simulink model "IndirectKalmanFilter"  (R2023b)
settings: Solver=ode4  StartTime=0.0  StopTime=2800  FixedStep=filter_Ts  RelTol=1e-3
InitFcn:
  | loadData;
values from neighbouring files (symbols this model uses):
  B_0 = Bk(x_0, imuSim.signals.values(1, 1:3)', imuSim.signals.values(1, 4:6)', filter_Ts)    [loadData.m]
  dx_0 = zeros(length(x_0), 1)    [loadData.m]
  F_0 = Fk(x_0, imuSim.signals.values(1, 1:3)', imuSim.signals.values(1, 4:6)', filter_Ts)    [loadData.m]
  filter_Ts = 0.01    [loadData.m]
  gps_sampling_time = 0.1    [loadData.m]
  imu_sampling_time = 0.01    [loadData.m]
  p_0 = 100 * eye(9)    [loadData.m]
  Qk = diag([1e-10, 1e-10, 1e-10, accel_var_continuous, gyro_var_continuous])    [computeImuProcessNoise.m]    (also in loadData.m = diag([1e-11, 1e-11, 1e-11, 4e-5,  4e-5,  4e-5, 1.2e-5, 1.2e-)
  Rk = diag([(7.84e-5)^2, (7.84e-5)^2, (2.0)^2, (0.1)^2, (0.1)^2, (0.1)^2])    [loadData.m]
  u_0 = imuSim.signals.values(1, :)    [loadData.m]
  x_0 = [lon_0;lat_0;h_0;vn_0;ve_0;vd_0;phi_0;theta_0;si_0]    [loadData.m]
libraries: simulink_extras x6, matrix_library x1
settings Model: Creator=amir  LastModifiedBy=amir

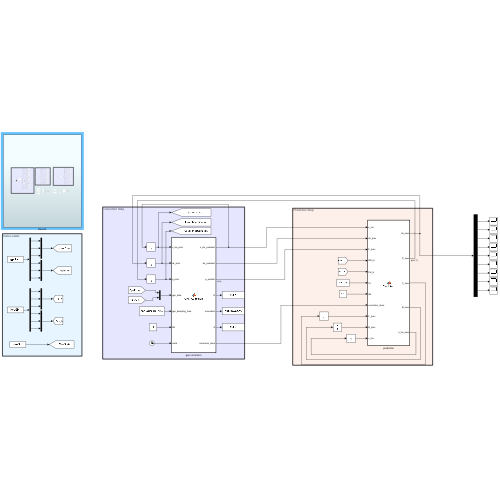
[thumbnail: Simulink's stored preview of the top-level diagram]
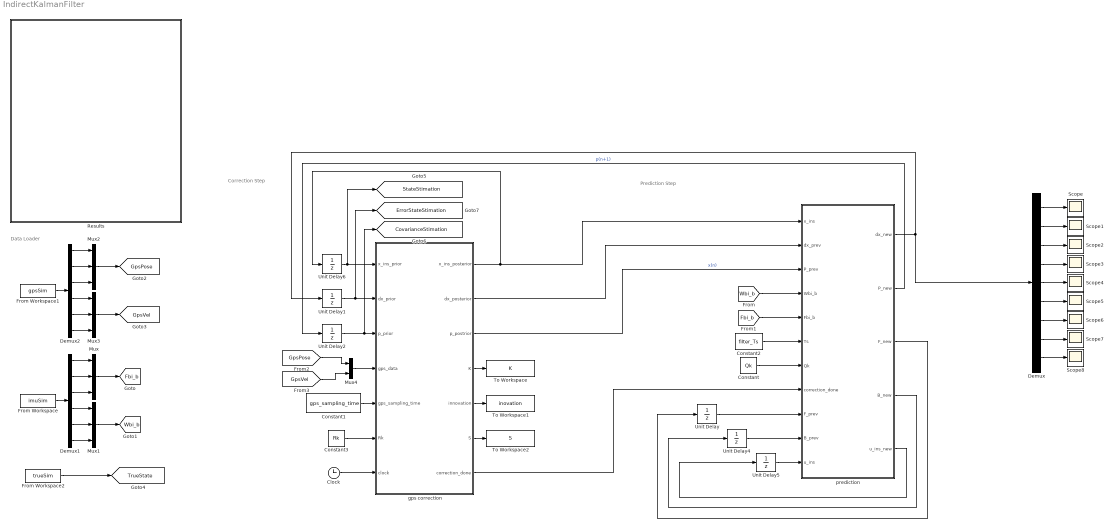
== system IndirectKalmanFilter ==
  note: Correction Step
  note: Data Loader
  note: Prediction Step
  Clock : Clock
  Constant : Constant  Value=Qk
  Constant1 : Constant  Value=gps_sampling_time
  Constant2 : Constant  Value=filter_Ts
  Constant3 : Constant  Value=Rk
  Demux : Demux  Outputs=9
  Demux1 : Demux  Outputs=6
  Demux2 : Demux  Outputs=6
  From Workspace : FromWorkspace  VariableName=imuSim  SampleTime=imu_sampling_time  Interpolate=off  OutputAfterFinalValue=Holding final value
  From Workspace1 : FromWorkspace  VariableName=gpsSim  SampleTime=gps_sampling_time  Interpolate=off  OutputAfterFinalValue=Holding final value
  From Workspace2 : FromWorkspace  VariableName=trueSim
  Mux{,1..3} (4 alike) : Mux  Inputs=3
  Mux4 : Mux  Inputs=2
  Results : Subsystem
  Scope{,1..8} (9 alike) : Scope
  To Workspace : ToWorkspace  VariableName=K  SampleTime=-1
  To Workspace1 : ToWorkspace  VariableName=inovation  SampleTime=-1
  To Workspace2 : ToWorkspace  VariableName=S  SampleTime=-1
  Unit Delay : UnitDelay  InitialCondition=F_0;  SampleTime=-1  HasFrameUpgradeWarning=on
  Unit Delay1 : UnitDelay  InitialCondition=dx_0;  SampleTime=-1  HasFrameUpgradeWarning=on
  Unit Delay2 : UnitDelay  InitialCondition=p_0;  SampleTime=-1  HasFrameUpgradeWarning=on
  Unit Delay4 : UnitDelay  InitialCondition=B_0;  SampleTime=-1  HasFrameUpgradeWarning=on
  Unit Delay5 : UnitDelay  InitialCondition=u_0';  SampleTime=-1  HasFrameUpgradeWarning=on
  Unit Delay6 : UnitDelay  InitialCondition=x_0;  SampleTime=-1  HasFrameUpgradeWarning=on
  gps correction : MATLAB Function  TreatAsAtomicUnit=on
  prediction : MATLAB Function  TreatAsAtomicUnit=on
  tag scope: CovarianceStimation=global, ErrorStateStimation=global, Fbi_b=global, GpsPose=global, GpsVel=global, StateStimation=global, TrueState=global, Wbi_b=global
  wires:
  Constant2/1 -> prediction/6(Ts)
  [Fbi_b] -> prediction/5(Fbi_b)
  [Wbi_b] -> prediction/4(Wbi_b)
  From Workspace/1 -> Demux1/1
  Demux1/2 -> Mux/2
  Demux1/3 -> Mux/3
  Demux1/4 -> Mux1/1
  Demux1/5 -> Mux1/2
  Demux1/6 -> Mux1/3
  Mux/1 -> [Fbi_b]
  Mux1/1 -> [Wbi_b]
  Demux1/1 -> Mux/1
  Demux2/1 -> Mux2/1
  Demux2/5 -> Mux3/2
  Demux2/6 -> Mux3/3
  Mux2/1 -> [GpsPose]
  Mux3/1 -> [GpsVel]
  Demux2/4 -> Mux3/1
  Demux2/3 -> Mux2/3
  Demux2/2 -> Mux2/2
  Constant/1 -> prediction/7(Qk)
  Clock/1 -> gps correction/7(clock)
  Constant1/1 -> gps correction/5(gps_sampling_time)
  Constant3/1 -> gps correction/6(Rk)
  [GpsPose] -> Mux4/1
  [GpsVel] -> Mux4/2
  Mux4/1 -> gps correction/4(gps_data)
  From Workspace2/1 -> [TrueState]
  From Workspace1/1 -> Demux2/1
  gps correction/4(K) -> To Workspace/1
  gps correction/6(S) -> To Workspace2/1
  gps correction/5(innovation) -> To Workspace1/1
  prediction/3(F_new) -> Unit Delay/1
  Unit Delay/1 -> prediction/9(F_prev)
  Unit Delay4/1 -> prediction/10(B_prev)
  prediction/4(B_new) -> Unit Delay4/1
  prediction/5(u_ins_new) -> Unit Delay5/1
  Unit Delay6/1 -> gps correction/1(x_ins_prior), [StateStimation]
  gps correction/1(x_ins_posterior) -> Unit Delay6/1, prediction/1(x_ins)
  Unit Delay5/1 -> prediction/11(u_ins)
  gps correction/3(p_postrior) -> prediction/3(P_prev)  "x(n)"
  gps correction/7(correction_done) -> prediction/8(correction_done)
  prediction/1(dx_new) -> Unit Delay1/1, Demux/1
  prediction/2(P_new) -> Unit Delay2/1  "p(n+1)"
  Unit Delay1/1 -> [ErrorStateStimation], gps correction/2(dx_prior)
  Unit Delay2/1 -> [CovarianceStimation], gps correction/3(p_prior)
  gps correction/2(dx_posterior) -> prediction/2(dx_prev)
  Demux/1 -> Scope/1
  Demux/2 -> Scope1/1
  Demux/3 -> Scope2/1
  Demux/4 -> Scope3/1
  Demux/5 -> Scope4/1
  Demux/6 -> Scope5/1
  Demux/7 -> Scope6/1
  Demux/8 -> Scope7/1
  Demux/9 -> Scope8/1

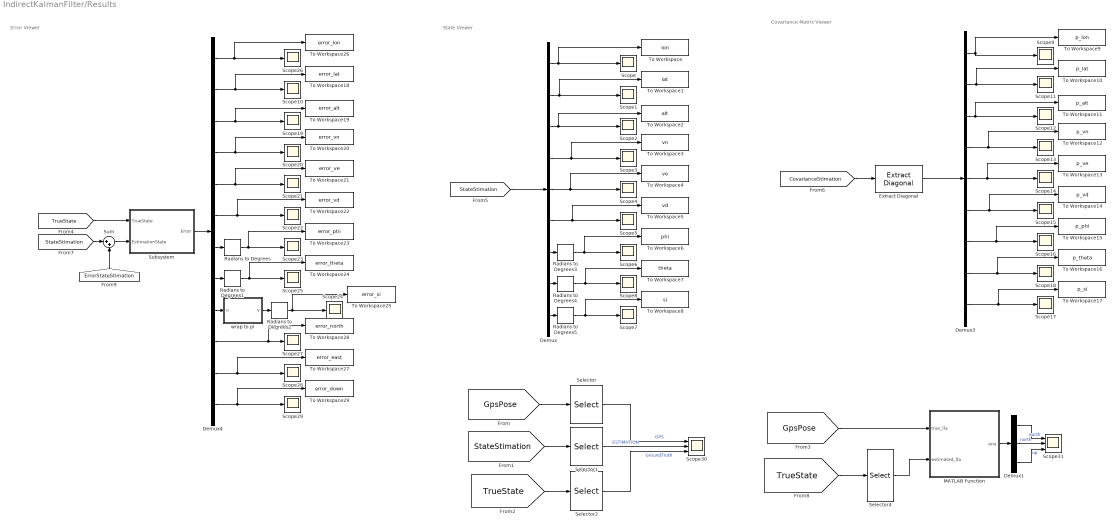
== system IndirectKalmanFilter/Results ==
  note: Error Viewer
  note: Covariance Matrix Viewer
  note: State Viewer
  Demux : Demux  Outputs=9
  Demux1 : Demux  Outputs=3
  Demux3 : Demux  Outputs=9
  Demux4 : Demux  Outputs=12
  Extract Diagonal : matrix_library/Extract Diagonal
      settings: LibrarySourceBlock=|
      | simulink/Matrix
      | Operations/Extract Diagonal
  MATLAB Function : MATLAB Function  TreatAsAtomicUnit=on
  Radians to Degrees{,1..5} (6 alike) : simulink_extras/Transformations/Radians to Degrees
  Scope{,1..29} (30 alike) : Scope
  Scope30 : Scope  NumInputPorts=3
  Scope31 : Scope  NumInputPorts=3
  Selector : Selector  InputPortWidth=3  IndexOptions=Index vector (dialog)  Indices=[3]  OutputSizes=1
  Selector1 : Selector  InputPortWidth=9  IndexOptions=Index vector (dialog)  Indices=[3]  OutputSizes=1
  Selector2 : Selector  InputPortWidth=9  IndexOptions=Index vector (dialog)  Indices=[3]  OutputSizes=1
  Selector4 : Selector  InputPortWidth=9  IndexOptions=Index vector (dialog)  Indices=[1 2 3]  OutputSizes=1
  Subsystem : Subsystem
  Sum : Sum  Inputs=|++
  To Workspace : ToWorkspace  VariableName=lon  SampleTime=-1
      settings: Save2DSignal=2-D array (concatenate along first dimension)
  To Workspace1 : ToWorkspace  VariableName=lat  SampleTime=-1
      settings: Save2DSignal=2-D array (concatenate along first dimension)
  To Workspace10 : ToWorkspace  VariableName=p_lat  SampleTime=-1
      settings: Save2DSignal=2-D array (concatenate along first dimension)
  To Workspace11 : ToWorkspace  VariableName=p_alt  SampleTime=-1
      settings: Save2DSignal=2-D array (concatenate along first dimension)
  To Workspace12 : ToWorkspace  VariableName=p_vn  SampleTime=-1
      settings: Save2DSignal=2-D array (concatenate along first dimension)
  To Workspace13 : ToWorkspace  VariableName=p_ve  SampleTime=-1
      settings: Save2DSignal=2-D array (concatenate along first dimension)
  To Workspace14 : ToWorkspace  VariableName=p_vd  SampleTime=-1
      settings: Save2DSignal=2-D array (concatenate along first dimension)
  To Workspace15 : ToWorkspace  VariableName=p_phi  SampleTime=-1
      settings: Save2DSignal=2-D array (concatenate along first dimension)
  To Workspace16 : ToWorkspace  VariableName=p_theta  SampleTime=-1
      settings: Save2DSignal=2-D array (concatenate along first dimension)
  To Workspace17 : ToWorkspace  VariableName=p_si  SampleTime=-1
      settings: Save2DSignal=2-D array (concatenate along first dimension)
  To Workspace18 : ToWorkspace  VariableName=error_lat  SampleTime=-1
      settings: Save2DSignal=2-D array (concatenate along first dimension)
  To Workspace19 : ToWorkspace  VariableName=error_alt  SampleTime=-1
      settings: Save2DSignal=2-D array (concatenate along first dimension)
  To Workspace2 : ToWorkspace  VariableName=alt  SampleTime=-1
      settings: Save2DSignal=2-D array (concatenate along first dimension)
  To Workspace20 : ToWorkspace  VariableName=error_vn  SampleTime=-1
      settings: Save2DSignal=2-D array (concatenate along first dimension)
  To Workspace21 : ToWorkspace  VariableName=error_ve  SampleTime=-1
      settings: Save2DSignal=2-D array (concatenate along first dimension)
  To Workspace22 : ToWorkspace  VariableName=error_vd  SampleTime=-1
      settings: Save2DSignal=2-D array (concatenate along first dimension)
  To Workspace23 : ToWorkspace  VariableName=error_phi  SampleTime=-1
      settings: Save2DSignal=2-D array (concatenate along first dimension)
  To Workspace24 : ToWorkspace  VariableName=error_theta  SampleTime=-1
      settings: Save2DSignal=2-D array (concatenate along first dimension)
  To Workspace25 : ToWorkspace  VariableName=error_si  SampleTime=-1
      settings: Save2DSignal=2-D array (concatenate along first dimension)
  To Workspace26 : ToWorkspace  VariableName=error_lon  SampleTime=-1
      settings: Save2DSignal=2-D array (concatenate along first dimension)
  To Workspace27 : ToWorkspace  VariableName=error_east  SampleTime=-1
      settings: Save2DSignal=2-D array (concatenate along first dimension)
  To Workspace28 : ToWorkspace  VariableName=error_north  SampleTime=-1
      settings: Save2DSignal=2-D array (concatenate along first dimension)
  To Workspace29 : ToWorkspace  VariableName=error_down  SampleTime=-1
      settings: Save2DSignal=2-D array (concatenate along first dimension)
  To Workspace3 : ToWorkspace  VariableName=vn  SampleTime=-1
      settings: Save2DSignal=2-D array (concatenate along first dimension)
  To Workspace4 : ToWorkspace  VariableName=ve  SampleTime=-1
      settings: Save2DSignal=2-D array (concatenate along first dimension)
  To Workspace5 : ToWorkspace  VariableName=vd  SampleTime=-1
      settings: Save2DSignal=2-D array (concatenate along first dimension)
  To Workspace6 : ToWorkspace  VariableName=phi  SampleTime=-1
      settings: Save2DSignal=2-D array (concatenate along first dimension)
  To Workspace7 : ToWorkspace  VariableName=theta  SampleTime=-1
      settings: Save2DSignal=2-D array (concatenate along first dimension)
  To Workspace8 : ToWorkspace  VariableName=si  SampleTime=-1
      settings: Save2DSignal=2-D array (concatenate along first dimension)
  To Workspace9 : ToWorkspace  VariableName=p_lon  SampleTime=-1
      settings: Save2DSignal=2-D array (concatenate along first dimension)
  wrap to pi : MATLAB Function  TreatAsAtomicUnit=on
  wires:
  Demux4/2 -> To Workspace18/1, Scope10/1
  Demux3/5 -> To Workspace13/1, Scope14/1
  Demux4/1 -> To Workspace26/1, Scope26/1
  Demux/6 -> To Workspace5/1, Scope5/1
  Demux/5 -> To Workspace4/1, Scope4/1
  Demux3/3 -> Scope12/1, To Workspace11/1
  Demux3/8 -> Scope18/1, To Workspace16/1
  Demux4/4 -> To Workspace20/1, Scope20/1
  Demux/4 -> To Workspace3/1, Scope3/1
  Demux/7 -> Radians to Degrees3/1
  Demux3/1 -> Scope9/1, To Workspace9/1
  Demux4/8 -> Radians to Degrees1/1
  Demux3/9 -> Scope17/1, To Workspace17/1
  Demux4/5 -> To Workspace21/1, Scope21/1
  Demux/1 -> Scope/1, To Workspace/1
  Demux4/3 -> To Workspace19/1, Scope19/1
  Demux3/7 -> Scope16/1, To Workspace15/1
  Demux3/6 -> To Workspace14/1, Scope15/1
  [StateStimation] -> Demux/1
  Demux/8 -> Radians to Degrees4/1
  Extract Diagonal/1 -> Demux3/1
  Demux4/6 -> To Workspace22/1, Scope22/1
  Demux4/7 -> Radians to Degrees/1
  Demux3/4 -> To Workspace12/1, Scope13/1
  Demux/9 -> Radians to Degrees5/1
  [CovarianceStimation] -> Extract Diagonal/1
  Demux/2 -> Scope1/1, To Workspace1/1
  Demux/3 -> Scope2/1, To Workspace2/1
  Demux3/2 -> Scope11/1, To Workspace10/1
  [TrueState] -> Subsystem/1(TrueState)
  Subsystem/1(Error) -> Demux4/1
  Demux4/10 -> To Workspace28/1, Scope27/1
  Demux4/11 -> To Workspace27/1, Scope28/1
  Demux4/12 -> Scope29/1, To Workspace29/1
  Radians to Degrees/1 -> Scope23/1, To Workspace23/1
  Radians to Degrees1/1 -> Scope25/1, To Workspace24/1
  Radians to Degrees2/1 -> Scope24/1, To Workspace25/1
  Radians to Degrees3/1 -> Scope6/1, To Workspace6/1
  Radians to Degrees4/1 -> Scope8/1, To Workspace7/1
  Radians to Degrees5/1 -> Scope7/1, To Workspace8/1
  [GpsPose] -> Selector/1
  [StateStimation] -> Selector1/1
  [TrueState] -> Selector2/1
  Selector/1 -> Scope30/1  "GPS"
  Selector1/1 -> Scope30/2  "ESTIMATION"
  Selector2/1 -> Scope30/3  "GroundTruth"
  Selector4/1 -> MATLAB Function/2(estimated_lla)
  [TrueState] -> Selector4/1
  MATLAB Function/1(enu) -> Demux1/1
  Demux1/1 -> Scope31/1  "earth"
  Demux1/2 -> Scope31/2  "north"
  Demux1/3 -> Scope31/3  "up"
  [GpsPose] -> MATLAB Function/1(true_lla)
  Demux4/9 -> wrap to pi/1(u)
  wrap to pi/1(y) -> Radians to Degrees2/1
  [StateStimation] -> Sum/1
  Sum/1 -> Subsystem/2(EstimationState)
  [ErrorStateStimation] -> Sum/2

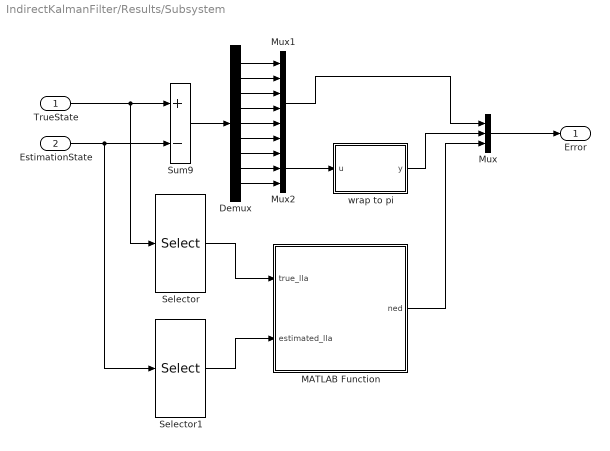
== system IndirectKalmanFilter/Results/Subsystem ==
  TrueState : Inport
  EstimationState : Inport  Port=2
  Demux : Demux  Outputs=9
  MATLAB Function : MATLAB Function  TreatAsAtomicUnit=on
  Mux : Mux  Inputs=3
  Mux1 : Mux  Inputs=6
  Mux2 : Mux  Inputs=3
  Selector : Selector  InputPortWidth=9  IndexOptions=Index vector (dialog)  Indices=[1 2 3]  OutputSizes=1
  Selector1 : Selector  InputPortWidth=9  IndexOptions=Index vector (dialog)  Indices=[1 2 3]  OutputSizes=1
  Sum9 : Sum  Inputs=+-
  wrap to pi : MATLAB Function  TreatAsAtomicUnit=on
  Error : Outport
  wires:
  TrueState/1 -> Selector/1, Sum9/1
  EstimationState/1 -> Selector1/1, Sum9/2
  Selector/1 -> MATLAB Function/1(true_lla)
  Selector1/1 -> MATLAB Function/2(estimated_lla)
  MATLAB Function/1(ned) -> Mux/3
  Mux/1 -> Error/1
  Sum9/1 -> Demux/1
  Demux/1 -> Mux1/1
  Demux/2 -> Mux1/2
  Demux/3 -> Mux1/3
  Demux/4 -> Mux1/4
  Demux/5 -> Mux1/5
  Demux/6 -> Mux1/6
  Demux/7 -> Mux2/1
  Demux/8 -> Mux2/2
  Demux/9 -> Mux2/3
  Mux1/1 -> Mux/1
  Mux2/1 -> wrap to pi/1(u)
  wrap to pi/1(y) -> Mux/2

== matlab function IndirectKalmanFilter/gps correction ==
  data: x_ins_posterior output; x_ins_prior input; dx_prior input; dx_posterior output; p_prior input; gps_data input; gps_sampling_time input; Rk input; p_postrior output; clock input; K output; innovation output; S output; correction_done output
function [x_ins_posterior, dx_posterior, p_postrior, K, innovation, S, correction_done] = GPS_Correction(x_ins_prior, dx_prior, p_prior, gps_data, gps_sampling_time, Rk, clock)
    coder.extrinsic('disp')
    p_postrior = p_prior;
    dx_posterior = dx_prior;
    x_ins_posterior = x_ins_prior;
    K = zeros(9, 7);
    innovation = zeros(7, 1); 
    S = zeros(7, 7);           
    correction_done = 0;

    if mod(clock, gps_sampling_time) == 0 
        vn = gps_data(4);
        ve = gps_data(5);
        sigma_vn2 = Rk(4,4);
        sigma_ve2 = Rk(5,5);
        denom = (vn^2 + ve^2)^2;
        sigma_si2 = (vn^2 * sigma_ve2 + ve^2 * sigma_vn2) / denom;
        si_meas = atan2(ve, vn);

        H = [eye(6), zeros(6,3);
             zeros(1,8), 1];
        
        S = H * p_prior * H' + blkdiag(Rk, sigma_si2);  
        dy = [gps_data; si_meas] - H * x_ins_prior;  
        K = p_prior * H' / S;  
        innovation = dy - H * dx_prior;


        dx_posterior = dx_prior + K * innovation;
        x_ins_posterior = x_ins_prior + dx_posterior;
        dx_posterior = zeros(length(dx_prior), 1);

        I = eye(9);
        p_postrior = (I - K * H) * p_prior * (I - K * H)' + K * blkdiag(Rk, sigma_si2) * K';

        correction_done = 1;
    end
end

== matlab function IndirectKalmanFilter/prediction ==
  data: x_ins input; dx_prev input; P_prev input; Wbi_b input; Fbi_b input; Ts input; Qk input; correction_done input; F_prev input; B_prev input; dx_new output; P_new output; F_new output; B_new output; u_ins input; u_ins_new output
function [dx_new, P_new, F_new, B_new, u_ins_new]  = Prediction(x_ins, dx_prev, P_prev, Wbi_b, Fbi_b, Ts, Qk, correction_done, F_prev, B_prev, u_ins)

    F_new = F_prev;
    B_new = B_prev;
    u_ins_new = u_ins;
    if correction_done
        u_ins_new = [Wbi_b; Fbi_b];
        F_new = Fk(x_ins, u_ins_new(1:3), u_ins_new(4:6), Ts);   
        B_new = Bk(x_ins, u_ins_new(1:3), u_ins_new(4:6), Ts);
    end
    
    dx_new = state_derivative(x_ins , u_ins_new(1:3), u_ins_new(4:6)) * Ts + F_new * dx_prev + B_new * ([Wbi_b; Fbi_b] - u_ins_new);
    P_new = F_new * P_prev * F_new.' + Qk;

end

== matlab function IndirectKalmanFilter/Results/Subsystem/MATLAB Function ==
  data: true_lla input; ned output; estimated_lla input
function ned = ned_distance(true_lla, estimated_lla)
    % true_lla, estimated_lla: [lat; lon; alt] in degrees, meters
    % enu: [east; north; up] in meters
    
    % Convert to radians
    lat0 = true_lla(1);
    lon0 = true_lla(2);
    
    % Convert both to ECEF
    ref_ecef = lla_to_ecef(true_lla);
    est_ecef = lla_to_ecef(estimated_lla);
    
    % Delta vector in ECEF
    d = est_ecef - ref_ecef;

        % Rotation matrix from ECEF to ENU
    T_NE = [-sin(lat0)*cos(lon0), -sin(lat0)*sin(lon0), cos(lat0);
            -sin(lon0),           cos(lon0),            0;
             -cos(lat0)*cos(lon0),  -cos(lat0)*sin(lon0), -sin(lat0)];
    
    % Convert ECEF delta to ENU
    ned = T_NE * d;
end

function ecef = lla_to_ecef(lla)
% Convert [lat; lon; alt] to ECEF
    lat = lla(1);
    lon = lla(2);
    alt = lla(3);

    % WGS84 ellipsoid parameters
    a = 6378137.0;                % semi-major axis
    f = 1 / 298.257223563;        % flattening
    e2 = f * (2 - f);             % eccentricity squared

    sin_lat = sin(lat);
    cos_lat = cos(lat);
    sin_lon = sin(lon);
    cos_lon = cos(lon);

    N = a / sqrt(1 - e2 * sin_lat^2);  % prime vertical radius

    x = (N + alt) * cos_lat * cos_lon;
    y = (N + alt) * cos_lat * sin_lon;
    z = (N * (1 - e2) + alt) * sin_lat;

    ecef = [x; y; z];
end

== matlab function IndirectKalmanFilter/Results/Subsystem/wrap to pi ==
  data: u input; y output
function y = wrap_to_pi(u)
    y = mod(u + pi, 2*pi) - pi;
end

== matlab function IndirectKalmanFilter/Results/MATLAB Function ==
  data: true_lla input; enu output; estimated_lla input
function enu = enu_distance(true_lla, estimated_lla)
    % true_lla, estimated_lla: [lat; lon; alt] in degrees, meters
    % enu: [east; north; up] in meters
    
    % Convert to radians
    lat0 = true_lla(1);
    lon0 = true_lla(2);
    
    % Convert both to ECEF
    ref_ecef = lla_to_ecef(true_lla);
    est_ecef = lla_to_ecef(estimated_lla);
    
    % Delta vector in ECEF
    d = est_ecef - ref_ecef;
    
    % Rotation matrix from ECEF to ENU
    R = [-sin(lon0),           cos(lon0),            0;
         -sin(lat0)*cos(lon0), -sin(lat0)*sin(lon0), cos(lat0);
          cos(lat0)*cos(lon0),  cos(lat0)*sin(lon0), sin(lat0)];
    
    % Convert ECEF delta to ENU
    enu = R * d;
end

function ecef = lla_to_ecef(lla)
% Convert [lat; lon; alt] to ECEF
    lat = lla(1);
    lon = lla(2);
    alt = lla(3);

    % WGS84 ellipsoid parameters
    a = 6378137.0;                % semi-major axis
    f = 1 / 298.257223563;        % flattening
    e2 = f * (2 - f);             % eccentricity squared

    sin_lat = sin(lat);
    cos_lat = cos(lat);
    sin_lon = sin(lon);
    cos_lon = cos(lon);

    N = a / sqrt(1 - e2 * sin_lat^2);  % prime vertical radius

    x = (N + alt) * cos_lat * cos_lon;
    y = (N + alt) * cos_lat * sin_lon;
    z = (N * (1 - e2) + alt) * sin_lat;

    ecef = [x; y; z];
end

== matlab function IndirectKalmanFilter/Results/wrap to pi ==
  data: u input; y output
function y = wrap_to_pi(u)
    y = mod(u + pi, 2*pi) - pi;
end
